simulink model "convinterleaver"  (Simulink 4.00)
settings: Solver=ode45  StartTime=0.0  StopTime=20  RelTol=1e-3
undefined symbols (not defined in the file): slcm
libraries: commcnvintrlv2 x2, simulink3 x1
settings Model: LastModifiedBy=agaltman  BlockReductionOpt=off

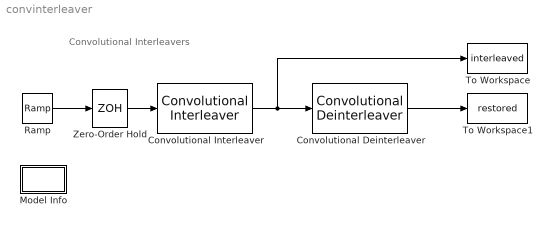
== system convinterleaver ==
  note: Convolutional Interleavers
  Convolutional Deinterleaver : commcnvintrlv2/Convolutional Deinterleaver  N=3  B=2  ic=[-1 -2 -3]'
  Convolutional Interleaver : commcnvintrlv2/Convolutional Interleaver  N=3  B=2  ic=[-1 -2 -3]'
  Model Info : Subsystem  LoadFcn=slcm LoadBlock;  InitFcn=slcm('UpdateAllCMBlocksInThisModelInit')  mask(CMBlock){InitialSaveTempField=, InitialBlockCM=none, BlockCM=none, Frame=on, SaveTempField=, DisplayStringWithTags=Info, MaskDisplayString=Info, HorizontalTextAlignment=Center, LeftAlignmentValue=0.5, SourceBlockDiagram=convinterleaver, TagMaxNumber=20, CMTag1=, CMTag2=, CMTag3=, CMTag4=, CMTag5=, CMTag6=, CMTag7=, CMTag8=, CMTag9=, CMTag10=, CMTag11=, CMTag12=, CMTag13=, CMTag14=, CMTag15=, CMTag16=, CMTag17=, CMTag18=, CMTag19=, CMTag20=}
      mask help: This block allows revision control information to be displayed within the model.
      settings: CopyFcn=slcm CopyBlock;  DeleteFcn=slcm Cancel;  PostSaveFcn=slcm('UpdateAllCMBlocksInThisModel')  NameChangeFcn=slcm Rename;  OpenFcn=commdemohelp;  RTWFcnNameOpts=Auto  RTWFileNameOpts=Auto
      mask Display: text(str2num(LeftAlignmentValue), 0.5, MaskDisplayString, 'HorizontalAlignment', HorizontalTextAlignment)
  Ramp : simulink3/Sources/Ramp  slope=1  start=0  X0=0
  To Workspace : ToWorkspace  VariableName=interleaved  SampleTime=-1  SaveFormat=Array
  To Workspace1 : ToWorkspace  VariableName=restored  SampleTime=-1  SaveFormat=Array
  Zero-Order Hold : ZeroOrderHold  SampleTime=1
  wires:
  Ramp/1 -> Zero-Order Hold/1
  Zero-Order Hold/1 -> Convolutional Interleaver/1
  Convolutional Interleaver/1 -> Convolutional Deinterleaver/1, To Workspace/1
  Convolutional Deinterleaver/1 -> To Workspace1/1

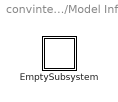
== system convinterleaver/Model Info ==
  EmptySubsystem : Subsystem
      settings: RTWFcnNameOpts=Auto  RTWFileNameOpts=Auto

== system convinterleaver/Model Info/EmptySubsystem ==
